simulink model "yin_2009_2"  (R2016a)
settings: Solver=VariableStepAuto  StartTime=0.0  StopTime=20  RelTol=1e-3
libraries: simulink x1
settings Model: Creator=M  LastModifiedBy=M

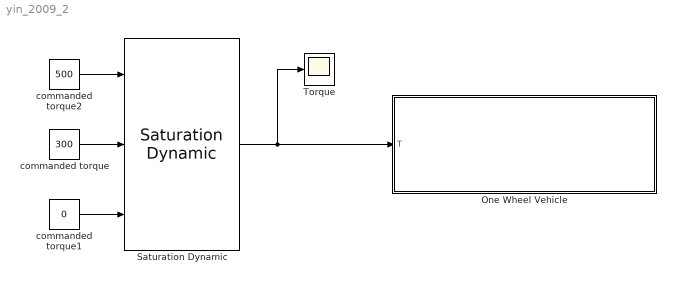
== system yin_2009_2 ==
  One Wheel Vehicle : Subsystem
  Saturation Dynamic : simulink/Discontinuities/Saturation Dynamic  OutMin=[]  OutMax=[]  OutDataTypeStr=Inherit: Same as second input  OutDataType=fixdt(1, 16)  OutScaling=2^-10  DoSatur=off
  Torque : Scope
  commanded torque : Constant  Value=300
  commanded torque1 : Constant  Value=0
  commanded torque2 : Constant  Value=500
  wires:
  Saturation Dynamic/1 -> Torque/1, One Wheel Vehicle/1(T)
  commanded torque/1 -> Saturation Dynamic/2
  commanded torque1/1 -> Saturation Dynamic/3
  commanded torque2/1 -> Saturation Dynamic/1

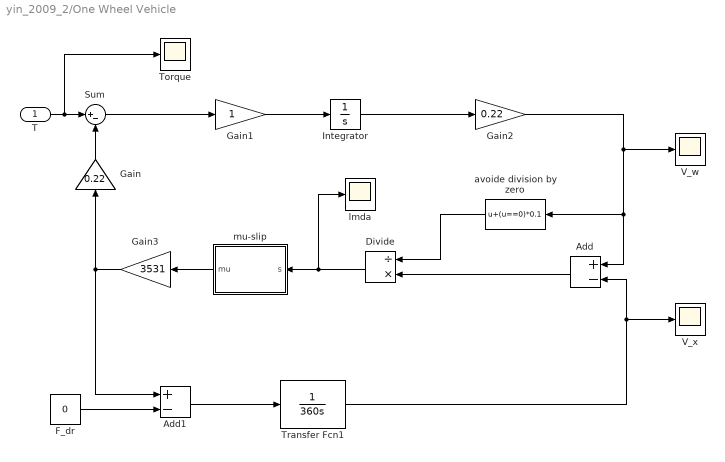
== system yin_2009_2/One Wheel Vehicle ==
  T : Inport
  " mu-slip" : MATLAB Function  TreatAsAtomicUnit=on
  Add : Sum  Inputs=+-
  Add1 : Sum  Inputs=+-
  Divide : Product  Inputs=/*
  F_dr : Constant  Value=0
  Gain : Gain  Gain=0.22
  Gain1 : Gain
  Gain2 : Gain  Gain=0.22
  Gain3 : Gain  Gain=3531
  Integrator : Integrator
  Sum : Sum  Inputs=|+-
  Torque : Scope
  Transfer Fcn1 : TransferFcn  Denominator=[360 0]
  V_w : Scope
  V_x : Scope
  avoide division by zero : MATLABFcn  MATLABFcn=u+(u==0)*0.1
  lmda : Scope
  wires:
  Gain/1 -> Sum/2
  Sum/1 -> Gain1/1
  Gain1/1 -> Integrator/1
  Gain3/1 -> Add1/1, Gain/1
  Add1/1 -> Transfer Fcn1/1
  Divide/1 -> " mu-slip"/1(s), lmda/1
  " mu-slip"/1(mu) -> Gain3/1
  F_dr/1 -> Add1/2
  Transfer Fcn1/1 -> V_x/1, Add/2
  Integrator/1 -> Gain2/1
  Add/1 -> Divide/2
  Gain2/1 -> avoide division by zero/1, Add/1, V_w/1
  T/1 -> Torque/1, Sum/1
  avoide division by zero/1 -> Divide/1

== matlab function yin_2009_2/One Wheel Vehicle/ mu-slip ==
  data: s input; mu output
function mu = fcn(s)

mu = sin(1.9 * atan(  10*s-0.97*(10*s-atan( 10*s )))  );
